simulink model "fwiine_example"  (Simulink 6.6)
settings: Solver=FixedStepDiscrete  StartTime=0.0  StopTime=100  FixedStep=0.1  MaxStep=0.5  RelTol=1e-3  SampleTimeConstraint=Specified
libraries: simulink x1
settings Model: Creator=William  LastModifiedBy=William
settings MATStruct: SampleTime=0.024  Offset=0  Priority=[10.0]
settings DataIOCC: MaxDataPoints=2500
settings DebuggingCC: AlgebraicLoopMsg=none  SolverPrmCheckMsg=none  UnconnectedInputMsg=none  UnconnectedOutputMsg=none  UnconnectedLineMsg=none
settings SimEventsCC: propLogEventsScheduled=0  propLogEventsExecuted=0  propLogDepartureEvents=0  propDisplayEventCalendar=0

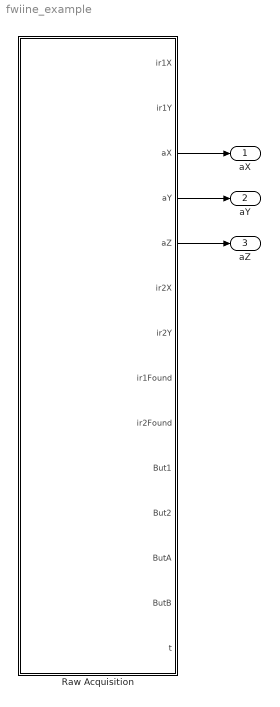
== system fwiine_example ==
  Raw Acquisition : Subsystem
  aX : Outport
  aY : Outport  Port=2
  aZ : Outport  Port=3
  wires:
  Raw Acquisition/3(aX) -> aX/1
  Raw Acquisition/4(aY) -> aY/1
  Raw Acquisition/5(aZ) -> aZ/1

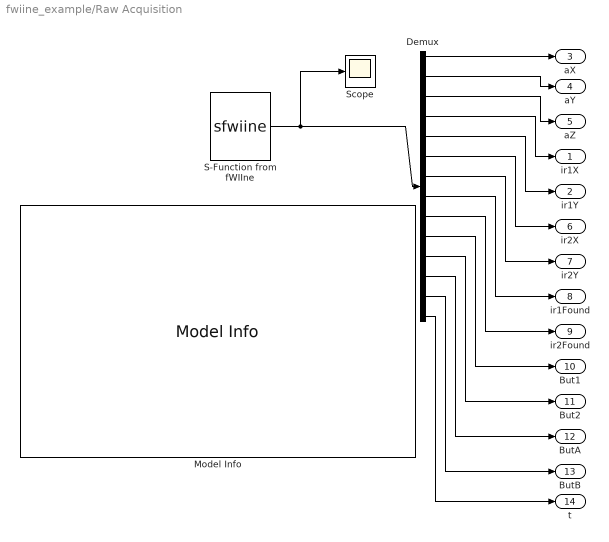
== system fwiine_example/Raw Acquisition ==
  Demux : Demux  Outputs=14
  Model Info : simulink/Model-Wide Utilities/Model Info  SystemSampleTime=-1  InitialBlockCM=None  BlockCM=None  Frame=on  DisplayStringWithTags=|  HorizontalTextAlignment=Left  LeftAlignmentValue=0.02  SourceBlockDiagram=fwiine_example  TagMaxNumber=20
      | S-function for fWIIne (Wiimote acquisition)
      | Filename : fwiine_example.mdl 
      | 
      | Date : 10/05/2008
      | Version : 0.2
      | Author : William Alozy
      | 
      | Comments :
      | 
      | To start with this unstable release :
      | - Set solver options type "Fixed-step", Solver "discrete (no continuous states)
      | - Set sample times properties "[[0.024,0,10];]", constraint "Specified"
  S-Function from fWIIne : S-Function  FunctionName=sfwiine
  Scope : Scope
      settings: TimeRange=100
  ir1X : Outport
  ir1Y : Outport  Port=2
  aX : Outport  Port=3
  aY : Outport  Port=4
  aZ : Outport  Port=5
  ir2X : Outport  Port=6
  ir2Y : Outport  Port=7
  ir1Found : Outport  Port=8
  ir2Found : Outport  Port=9
  But1 : Outport  Port=10
  But2 : Outport  Port=11
  ButA : Outport  Port=12
  ButB : Outport  Port=13
  t : Outport  Port=14
  wires:
  S-Function from fWIIne/1 -> Demux/1, Scope/1
  Demux/1 -> aX/1
  Demux/2 -> aY/1
  Demux/3 -> aZ/1
  Demux/4 -> ir1X/1
  Demux/5 -> ir1Y/1
  Demux/6 -> ir2X/1
  Demux/8 -> ir1Found/1
  Demux/9 -> ir2Found/1
  Demux/10 -> But1/1
  Demux/11 -> But2/1
  Demux/12 -> ButA/1
  Demux/13 -> ButB/1
  Demux/7 -> ir2Y/1
  Demux/14 -> t/1
